simulink model "reducedorderobserver"  (R2023a)
settings: Solver=VariableStepAuto  StartTime=0.0  StopTime=10.0  RelTol=1e-3
undefined symbols (not defined in the file): A_aa_disc, A_ab_disc, A_ba_disc, A_bb_disc, absolute_encoder_counts_per_revolution, B_a_disc, B_b_disc, DiscIntNeverNeededParam, g, gyro_sigma_drift, I_noload, init, K_disc_int, K_disc_x, K_m, l, L_r_disc, m, min_sampling_time, potentiometer_linearity_percent, R, sys_disc, theta_l_init, vision_fps, x1_bar, x2_bar
settings Model: Creator=yunzh  LastModifiedBy=yunzh

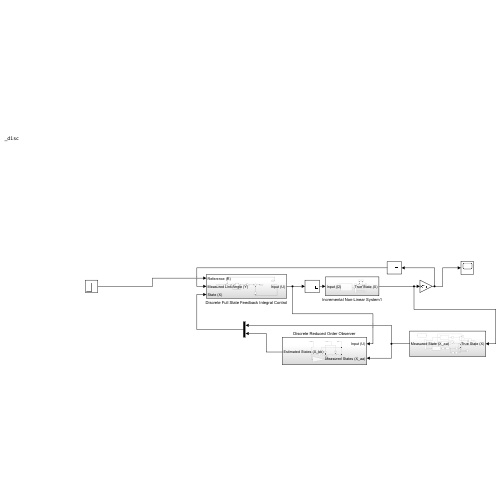
[thumbnail: Simulink's stored preview of the top-level diagram]
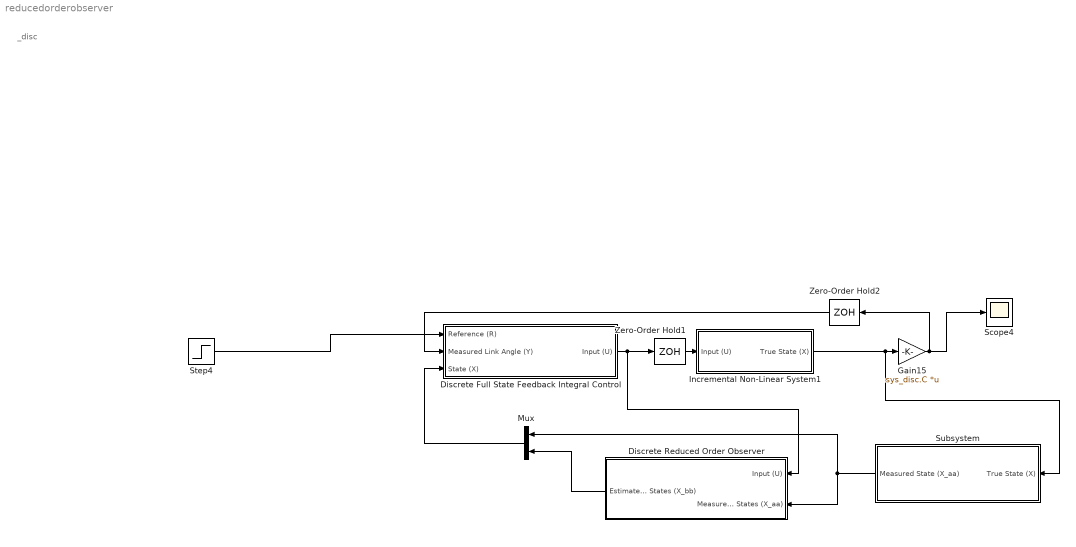
== system reducedorderobserver ==
  note: _disc
  Discrete Full State Feedback Integral Control : Subsystem
  Discrete Reduced Order Observer : Subsystem
  Gain15 : Gain  Gain=sys_disc.C  Multiplication=Matrix(K*u)
  Incremental Non-Linear System1 : Subsystem
  Mux : Mux  Inputs=2
  Scope4 : Scope
  Step4 : Step  Time=0  After=deg2rad(15)  SampleTime=min_sampling_time
  Subsystem : Subsystem
  Zero-Order Hold1 : ZeroOrderHold  SampleTime=min_sampling_time
  Zero-Order Hold2 : ZeroOrderHold  SampleTime=min_sampling_time
  wires:
  Incremental Non-Linear System1/1(True State (X)) -> Subsystem/1(True State (X)), Gain15/1
  Step4/1 -> Discrete Full State Feedback Integral Control/1(Reference (R))
  Gain15/1 -> Zero-Order Hold2/1, Scope4/1
  Discrete Full State Feedback Integral Control/1(Input (U)) -> Discrete Reduced Order Observer/1(Input (U)), Zero-Order Hold1/1
  Zero-Order Hold1/1 -> Incremental Non-Linear System1/1(Input (U))
  Discrete Reduced Order Observer/1(Estimated States (X_bb)) -> Mux/2
  Mux/1 -> Discrete Full State Feedback Integral Control/3(State (X))
  Zero-Order Hold2/1 -> Discrete Full State Feedback Integral Control/2(Measured Link Angle (Y))
  Subsystem/1(Measured State (X_aa)) -> Discrete Reduced Order Observer/2(Measured States (X_aa)), Mux/1

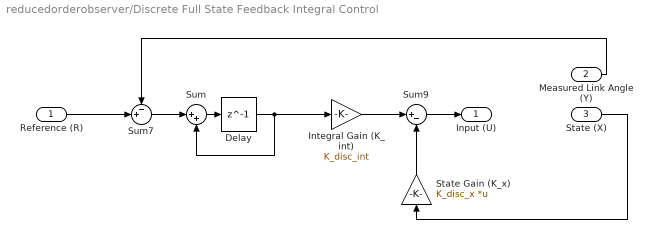
== system reducedorderobserver/Discrete Full State Feedback Integral Control ==
  Reference (R) : Inport
  Measured Link Angle (Y) : Inport  Port=2
  State (X) : Inport  Port=3
  Delay : Delay  DelayLength=1  SampleTime=min_sampling_time
  Integral Gain (K_int) : Gain  Gain=K_disc_int
  State Gain (K_x) : Gain  Gain=K_disc_x  Multiplication=Matrix(K*u)
  Sum : Sum  Inputs=|++
  Sum7 : Sum  Inputs=-+|
  Sum9 : Sum  Inputs=|+-
  Input (U) : Outport
  wires:
  Integral Gain (K_int)/1 -> Sum9/1
  Reference (R)/1 -> Sum7/2
  Sum/1 -> Delay/1
  State Gain (K_x)/1 -> Sum9/2
  Sum7/1 -> Sum/1
  Delay/1 -> Sum/2, Integral Gain (K_int)/1
  Sum9/1 -> Input (U)/1
  State (X)/1 -> State Gain (K_x)/1
  Measured Link Angle (Y)/1 -> Sum7/1

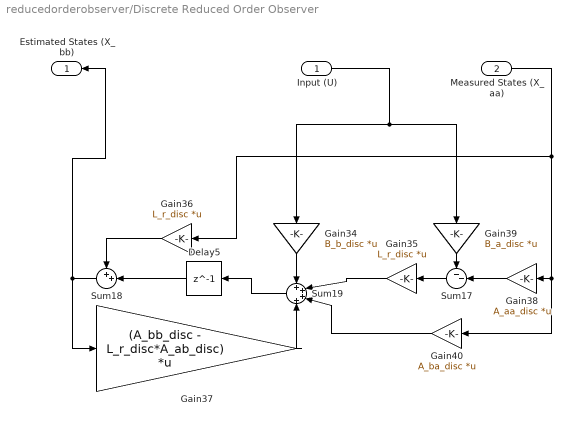
== system reducedorderobserver/Discrete Reduced Order Observer ==
  Input (U) : Inport
  Measured States (X_aa) : Inport  Port=2
  Delay5 : Delay  DelayLength=1  SampleTime=min_sampling_time
  Gain34 : Gain  Gain=B_b_disc  Multiplication=Matrix(K*u)
  Gain35 : Gain  Gain=L_r_disc  Multiplication=Matrix(K*u)
  Gain36 : Gain  Gain=L_r_disc  Multiplication=Matrix(K*u)
  Gain37 : Gain  Gain=(A_bb_disc - L_r_disc*A_ab_disc)  Multiplication=Matrix(K*u)
  Gain38 : Gain  Gain=A_aa_disc  Multiplication=Matrix(K*u)
  Gain39 : Gain  Gain=B_a_disc  Multiplication=Matrix(K*u)
  Gain40 : Gain  Gain=A_ba_disc  Multiplication=Matrix(K*u)
  Sum17 : Sum  Inputs=--|
  Sum18 : Sum  Inputs=++|
  Sum19 : Sum  Inputs=++++
  Estimated States (X_bb) : Outport
  wires:
  Gain40/1 -> Sum19/3
  Gain35/1 -> Sum19/2
  Gain37/1 -> Sum19/4
  Measured States (X_aa)/1 -> Gain38/1, Gain40/1, Gain36/1
  Gain34/1 -> Sum19/1
  Delay5/1 -> Sum18/2
  Sum17/1 -> Gain35/1
  Gain38/1 -> Sum17/2
  Sum19/1 -> Delay5/1
  Sum18/1 -> Estimated States (X_bb)/1, Gain37/1
  Gain36/1 -> Sum18/1
  Gain39/1 -> Sum17/1
  Input (U)/1 -> Gain39/1, Gain34/1

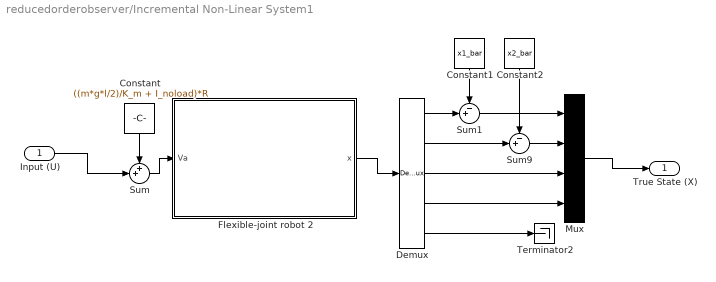
== system reducedorderobserver/Incremental Non-Linear System1 ==
  Input (U) : Inport
  Constant : Constant  Value=((m*g*l/2)/K_m + I_noload)*R
  Constant1 : Constant  Value=x1_bar
  Constant2 : Constant  Value=x2_bar
  Demux : Demux  Outputs=5
  Flexible-joint robot 2 : Subsystem
      mask Display: image('$imagefile'); % Use "Edit Image" on toolstrip to change.
  Mux : Mux
  Sum : Sum  Inputs=++|
  Sum1 : Sum  Inputs=-+|
  Sum9 : Sum  Inputs=-+|
  Terminator2 : Terminator
  True State (X) : Outport
  wires:
  Flexible-joint robot 2/1(x) -> Demux/1
  Demux/1 -> Sum1/2
  Demux/2 -> Sum9/2
  Demux/5 -> Terminator2/1
  Sum/1 -> Flexible-joint robot 2/1(Va)
  Constant1/1 -> Sum1/1
  Sum9/1 -> Mux/2
  Constant2/1 -> Sum9/1
  Sum1/1 -> Mux/1
  Demux/4 -> Mux/4
  Demux/3 -> Mux/3
  Constant/1 -> Sum/1
  Input (U)/1 -> Sum/2
  Mux/1 -> True State (X)/1

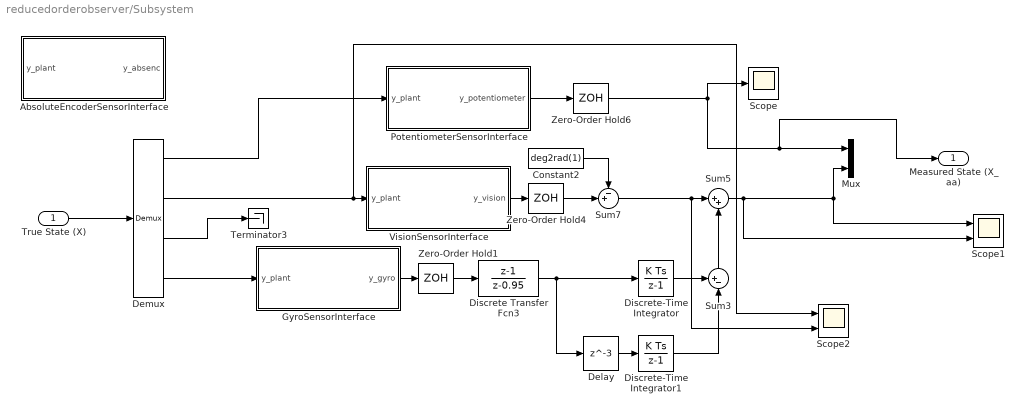
== system reducedorderobserver/Subsystem ==
  True State (X) : Inport
  AbsoluteEncoderSensorInterface : Subsystem  TreatAsAtomicUnit=on
      mask Display: image('$imagefile'); % Use "Edit Image" on toolstrip to change.
  Constant2 : Constant  Value=deg2rad(1)
  Delay : Delay  DelayLength=3  InitialCondition=0  SampleTime=min_sampling_time
  Demux : Demux
  Discrete Transfer Fcn3 : DiscreteTransferFcn  Numerator=[1 -1]  Denominator=[1 -0.95]  SampleTime=min_sampling_time
  Discrete-Time Integrator : DiscreteIntegrator  InitialCondition=theta_l_init  SampleTime=min_sampling_time  ICPrevOutput=DiscIntNeverNeededParam  ICPrevScaledInput=DiscIntNeverNeededParam
  Discrete-Time Integrator1 : DiscreteIntegrator  InitialCondition=theta_l_init  SampleTime=min_sampling_time  ICPrevOutput=DiscIntNeverNeededParam  ICPrevScaledInput=DiscIntNeverNeededParam
  GyroSensorInterface : Subsystem  TreatAsAtomicUnit=on
      mask Display: image('$imagefile'); % Use "Edit Image" on toolstrip to change.
  Mux : Mux  Inputs=2
  PotentiometerSensorInterface : Subsystem  TreatAsAtomicUnit=on
      mask Display: image('$imagefile'); % Use "Edit Image" on toolstrip to change.
  Scope : Scope
  Scope1 : Scope  NumInputPorts=2
  Scope2 : Scope  NumInputPorts=2
  Sum3 : Sum  Inputs=+-|
  Sum5 : Sum  Inputs=|++
  Sum7 : Sum  Inputs=-+|
  Terminator3 : Terminator
  VisionSensorInterface : Subsystem  TreatAsAtomicUnit=on
      mask Display: image('$imagefile'); % Use "Edit Image" on toolstrip to change.
  Zero-Order Hold1 : ZeroOrderHold  SampleTime=min_sampling_time
  Zero-Order Hold4 : ZeroOrderHold  SampleTime=min_sampling_time
  Zero-Order Hold6 : ZeroOrderHold  SampleTime=min_sampling_time
  Measured State (X_aa) : Outport
  wires:
  Discrete Transfer Fcn3/1 -> Delay/1, Discrete-Time Integrator/1
  Sum3/1 -> Sum5/2
  Sum7/1 -> Scope2/2, Sum5/1
  Delay/1 -> Discrete-Time Integrator1/1
  Constant2/1 -> Sum7/1
  Discrete-Time Integrator/1 -> Sum3/1
  Discrete-Time Integrator1/1 -> Sum3/2
  VisionSensorInterface/1(y_vision) -> Zero-Order Hold4/1
  Demux/3 -> Terminator3/1
  PotentiometerSensorInterface/1(y_potentiometer) -> Zero-Order Hold6/1
  GyroSensorInterface/1(y_gyro) -> Zero-Order Hold1/1
  Zero-Order Hold1/1 -> Discrete Transfer Fcn3/1
  Demux/4 -> GyroSensorInterface/1(y_plant)
  Demux/2 -> Scope2/1, VisionSensorInterface/1(y_plant)
  Zero-Order Hold4/1 -> Sum7/2
  Demux/1 -> PotentiometerSensorInterface/1(y_plant)
  Zero-Order Hold6/1 -> Scope/1, Measured State (X_aa)/1, Mux/1
  True State (X)/1 -> Demux/1
  Sum5/1 -> Scope1/1, Mux/2, Scope1/2

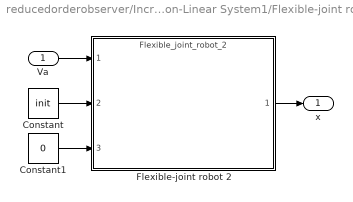
== system reducedorderobserver/Incremental Non-Linear System1/Flexible-joint robot 2 ==
  Va : Inport
  Constant : Constant  Value=init
  Constant1 : Constant  Value=0
  Flexible-joint robot 2 : ModelReference  ModelNameDialog=Flexible_joint_robot_2  ModelReferenceVersion=1.65  CopyOfModelProtected=on
  x : Outport
  wires:
  Va/1 -> Flexible-joint robot 2/1
  Constant1/1 -> Flexible-joint robot 2/3
  Constant/1 -> Flexible-joint robot 2/2
  Flexible-joint robot 2/1 -> x/1

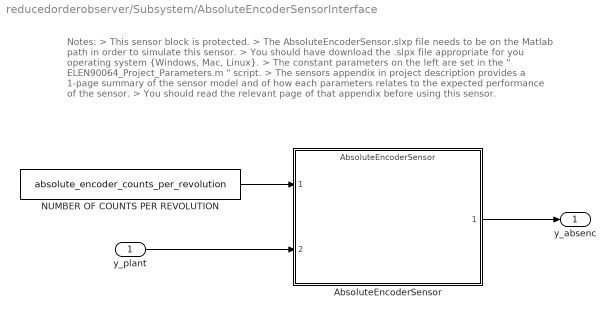
== system reducedorderobserver/Subsystem/AbsoluteEncoderSensorInterface ==
  note: Notes:
      | > This sensor block is protected.
      | > The AbsoluteEncoderSensor.slxp file needs to be on the Matlab path in order to simulate this sensor.
      | > You should have download the .slpx file appropriate for you operating system {Windows, Mac, Linux}.
      | > The constant parameters on the left are set in the " ELEN90064_Project_Parameters.m " script.
      | > The sensors appendix in project description provides a 1-page summary of the sensor model and of how each parameters relates to the expected performance of the sensor.
      | > You should read the relevant page of that appendix before using this sensor.
  y_plant : Inport
  AbsoluteEncoderSensor : ModelReference  ModelNameDialog=AbsoluteEncoderSensor.slxp  ModelReferenceVersion=1.16  CopyOfModelProtected=on
  NUMBER OF COUNTS PER REVOLUTION : Constant  Value=absolute_encoder_counts_per_revolution
  y_absenc : Outport
  wires:
  NUMBER OF COUNTS PER REVOLUTION/1 -> AbsoluteEncoderSensor/1
  y_plant/1 -> AbsoluteEncoderSensor/2
  AbsoluteEncoderSensor/1 -> y_absenc/1

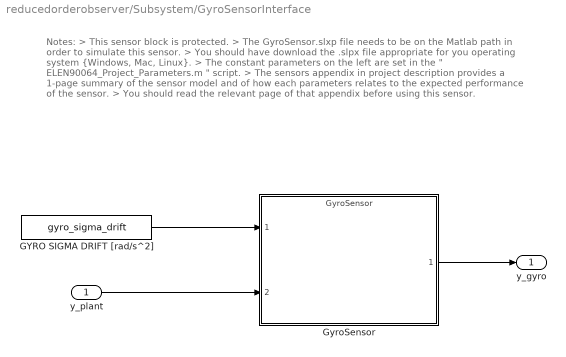
== system reducedorderobserver/Subsystem/GyroSensorInterface ==
  note: Notes:
      | > This sensor block is protected.
      | > The GyroSensor.slxp file needs to be on the Matlab path in order to simulate this sensor.
      | > You should have download the .slpx file appropriate for you operating system {Windows, Mac, Linux}.
      | > The constant parameters on the left are set in the " ELEN90064_Project_Parameters.m " script.
      | > The sensors appendix in project description provides a 1-page summary of the sensor model and of how each parameters relates to the expected performance of the sensor.
      | > You should read the relevant page of that appendix before using this sensor.
  y_plant : Inport
  GYRO SIGMA DRIFT [rad/s^2] : Constant  Value=gyro_sigma_drift
  GyroSensor : ModelReference  ModelNameDialog=GyroSensor.slxp  ModelReferenceVersion=1.18  CopyOfModelProtected=on
  y_gyro : Outport
  wires:
  GYRO SIGMA DRIFT [rad/s^2]/1 -> GyroSensor/1
  y_plant/1 -> GyroSensor/2
  GyroSensor/1 -> y_gyro/1

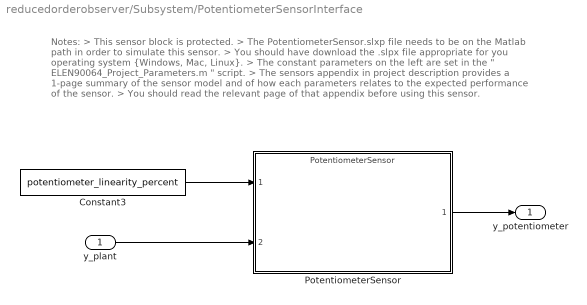
== system reducedorderobserver/Subsystem/PotentiometerSensorInterface ==
  note: Notes:
      | > This sensor block is protected.
      | > The PotentiometerSensor.slxp file needs to be on the Matlab path in order to simulate this sensor.
      | > You should have download the .slpx file appropriate for you operating system {Windows, Mac, Linux}.
      | > The constant parameters on the left are set in the " ELEN90064_Project_Parameters.m " script.
      | > The sensors appendix in project description provides a 1-page summary of the sensor model and of how each parameters relates to the expected performance of the sensor.
      | > You should read the relevant page of that appendix before using this sensor.
  y_plant : Inport
  Constant3 : Constant  Value=potentiometer_linearity_percent
  PotentiometerSensor : ModelReference  ModelNameDialog=PotentiometerSensor.slxp  ModelReferenceVersion=1.21  CopyOfModelProtected=on
  y_potentiometer : Outport
  wires:
  y_plant/1 -> PotentiometerSensor/2
  Constant3/1 -> PotentiometerSensor/1
  PotentiometerSensor/1 -> y_potentiometer/1

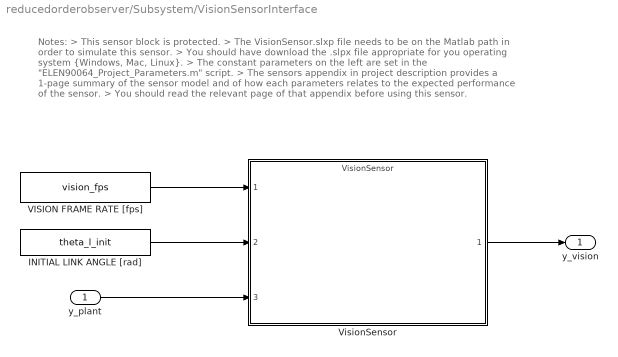
== system reducedorderobserver/Subsystem/VisionSensorInterface ==
  note: Notes:
      | > This sensor block is protected.
      | > The VisionSensor.slxp file needs to be on the Matlab path in order to simulate this sensor.
      | > You should have download the .slpx file appropriate for you operating system {Windows, Mac, Linux}.
      | > The constant parameters on the left are set in the "ELEN90064_Project_Parameters.m" script.
      | > The sensors appendix in project description provides a 1-page summary of the sensor model and of how each parameters relates to the expected performance of the sensor.
      | > You should read the relevant page of that appendix before using this sensor.
  y_plant : Inport
  INITIAL LINK ANGLE [rad] : Constant  Value=theta_l_init
  VISION FRAME RATE [fps] : Constant  Value=vision_fps
  VisionSensor : ModelReference  ModelNameDialog=VisionSensor.slxp  ModelReferenceVersion=1.19  CopyOfModelProtected=on
  y_vision : Outport
  wires:
  VISION FRAME RATE [fps]/1 -> VisionSensor/1
  INITIAL LINK ANGLE [rad]/1 -> VisionSensor/2
  y_plant/1 -> VisionSensor/3
  VisionSensor/1 -> y_vision/1
